simulink model "bf_swarm_generated"  (R2025a)
settings: Solver=ode4  StartTime=0.0  StopTime=60  FixedStep=0.002  RelTol=1e-3
model workspace (MAT data in the model file):
  cfg.N = 3
  cfg.mode = 'paper'
  cfg.T = 60
  cfg.dt = 0.002
  cfg.Ts = 0.01
  cfg.logTs = 0.02
  cfg.visualTs = 0.05
  cfg.visualize = 1
  cfg.pacing = 0
  cfg.receiver = [4; -3; 15]
  cfg.radius = 0.8
  cfg.path.center = [0; 0; 3]
  cfg.path.amplitude = [2.5; 1.5; 0.35]
  cfg.path.period = 40
  cfg.path.ramp = 5
  cfg.path.type = 'figure8'
  cfg.frameSeed = [1; 0; 0]
  cfg.yaw = 0
  cfg.initial.centroidError = [0.15; -0.1; 0.1]
  cfg.initial.formationRotation = [0; 0.209439510239; 0]
  cfg.initial.individualError = 0
  cfg.control.Kp = [2.5; 2.5; 3.5]
  cfg.control.Kd = [2.8; 2.8; 3.2]
  cfg.control.beta = 1.3
  cfg.control.kc = 0.9
  cfg.control.kv = 0.45
  cfg.control.ka = 3.2
  cfg.control.kq = 1
  cfg.control.kPlane = 4
  cfg.control.dPlane = 3
  cfg.control.maxHorizontalAccel = 4
  cfg.control.maxVerticalAccel = 4
  cfg.control.maxTilt = 0.610865238198
  cfg.vehicle.mass = 1
  cfg.vehicle.g = 9.81
  cfg.vehicle.I = [0.015  0  0; 0  0.015  0; 0  0  0.025]
  cfg.vehicle.arm = 0.225
  cfg.vehicle.kT = 1.8e-05
  cfg.vehicle.kQ = 2.7e-07
  cfg.vehicle.motorTau = 0.025
  cfg.vehicle.omegaMax = 620
  cfg.vehicle.drag = [0.12; 0.12; 0.18]
  cfg.vehicle.angularDrag = [0.002; 0.002; 0.003]
  cfg.vehicle.KR = [2.2; 2.2; 1.2]
  cfg.vehicle.Kw = [0.32; 0.32; 0.28]
  cfg.vehicle.bodyRadius = 0.27
  cfg.vehicle.rotorXY = [0.159099025767  -0.159099025767  -0.159099025767  0.159099025767; 0.159099025767  0.159099025767  -0.159099025767  -0.159099025767]
  cfg.vehicle.spin = [1 -1 1 -1]
  cfg.vehicle.B = [1  1  1  1; 0.159099025767  0.159099025767  -0.159099025767  -0.159099025767; -0.159099025767  0.159099025767  0.159099025767  -0.159099025767; 0.015  -0.015  0.015  -0.015]
  cfg.vehicle.Binv = [0.25  1.57134840264  -1.57134840264  16.6666666667; 0.25  1.57134840264  1.57134840264  -16.6666666667; 0.25  -1.57134840264  1.57134840264  16.6666666667; 0.25  -1.57134840264  -1.57134840264  -16.6666666667]
  cfg.vehicle.fMax = 6.9192
  cfg.wind.enabled = 0
  cfg.wind.velocity = [0.8; 0.3; 0]
  cfg.wind.gust = [0.3; 0.2; 0.1]
  cfg.rf.frequency = 138000000
  cfg.rf.c = 299792458
  cfg.rf.powerPerDrone = 0.1
  cfg.rf.noisePower = 1e-13
  cfg.rf.phaseOffsets = [0; 0; 0]
  cfg.rf.enabled = 1
  cfg.rho = [0.8  -0.4  -0.4; 0  0.692820323028  -0.692820323028; 0  0  0]
  cfg.edges = [1  2; 1  3; 2  3]
  cfg.edgeLength = [1.38564064606; 1.38564064606; 1.38564064606]
  cfg.minSeparation = 0.54
  cfg.lambda = 2.17240911594
  cfg.x0 = [0.844904723425  -0.162516209726  -0.232388513699; -0.040298923068  0.542283901867  -0.801984978799; 2.70815410328  3.4602846209  3.13156127581; 0  0  0; 0  0  0; 0  0  0; 1  1  1; 0  0  0; 0  0  0; 0  0  0; 0  0  0; 0  0  0; 0  0  0; 369.120576506  369.120576506  369.120576506; 369.120576506  369.120576506  369.120576506; 369.120576506  369.120576506  369.120576506; 369.120576506  369.120576506  369.120576506]
settings Model: Creator=Pranav R  LastModifiedBy=Pranav R
settings DataIOCC: SaveOutput=off  SignalLogging=off  SaveTime=off

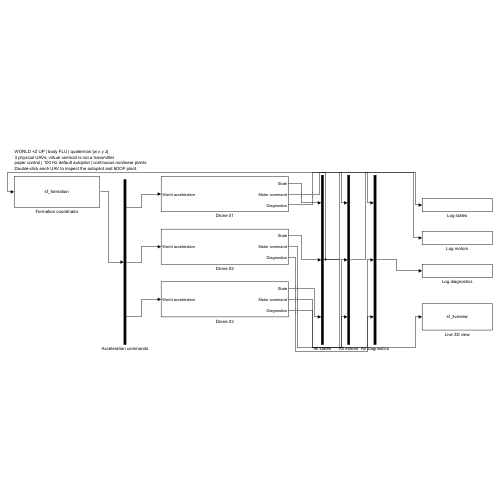
[thumbnail: Simulink's stored preview of the top-level diagram]
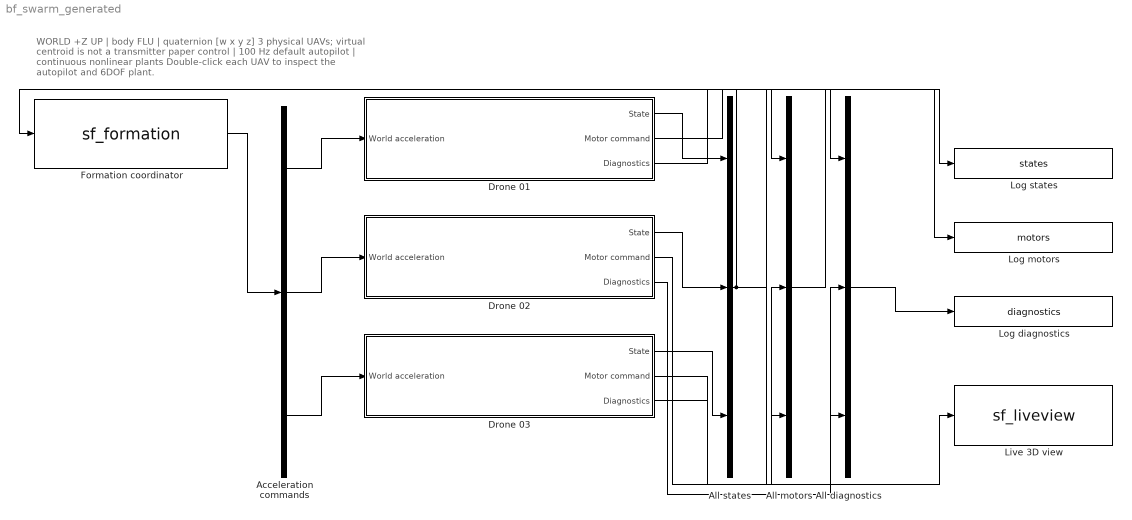
== system bf_swarm_generated ==
  note: WORLD +Z UP | body FLU | quaternion [w x y z]
      | 3 physical UAVs; virtual centroid is not a transmitter
      | paper control | 100 Hz default autopilot | continuous nonlinear plants
      | Double-click each UAV to inspect the autopilot and 6DOF plant.
  Acceleration commands : Demux  Outputs=[3 3 3]
  All diagnostics : Mux  Inputs=3
  All motors : Mux  Inputs=3
  All states : Mux  Inputs=3
  Drone 01 : Subsystem
  Drone 02 : Subsystem
  Drone 03 : Subsystem
  Formation coordinator : M-S-Function  FunctionName=sf_formation  Parameters=cfg
  Live 3D view : M-S-Function  FunctionName=sf_liveview  Parameters=cfg
  Log diagnostics : ToWorkspace  VariableName=diagnostics  SaveFormat=Timeseries  SampleTime=cfg.logTs
  Log motors : ToWorkspace  VariableName=motors  SaveFormat=Timeseries  SampleTime=cfg.logTs
  Log states : ToWorkspace  VariableName=states  SaveFormat=Timeseries  SampleTime=cfg.logTs
  wires:
  Formation coordinator/1 -> Acceleration commands/1
  Acceleration commands/1 -> Drone 01/1(World acceleration)
  Drone 01/1(State) -> All states/1
  Drone 01/2(Motor command) -> All motors/1
  Drone 01/3(Diagnostics) -> All diagnostics/1
  Acceleration commands/2 -> Drone 02/1(World acceleration)
  Drone 02/1(State) -> All states/2
  Drone 02/2(Motor command) -> All motors/2
  Drone 02/3(Diagnostics) -> All diagnostics/2
  Acceleration commands/3 -> Drone 03/1(World acceleration)
  Drone 03/1(State) -> All states/3
  Drone 03/2(Motor command) -> All motors/3
  Drone 03/3(Diagnostics) -> All diagnostics/3
  All states/1 -> Formation coordinator/1, Log states/1, Live 3D view/1
  All motors/1 -> Log motors/1
  All diagnostics/1 -> Log diagnostics/1

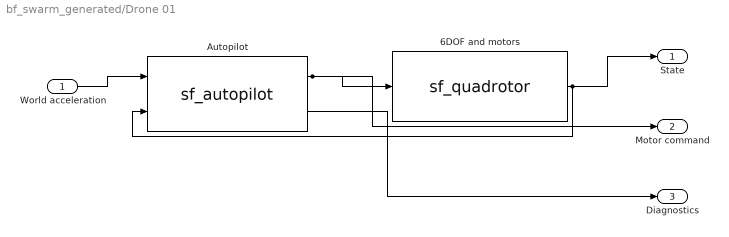
== system bf_swarm_generated/Drone 01 ==
  World acceleration : Inport
  6DOF and motors : M-S-Function  FunctionName=sf_quadrotor  Parameters=cfg,1
  Autopilot : M-S-Function  FunctionName=sf_autopilot  Parameters=cfg
  State : Outport
  Motor command : Outport  Port=2
  Diagnostics : Outport  Port=3
  wires:
  World acceleration/1 -> Autopilot/1
  Autopilot/1 -> 6DOF and motors/1, Motor command/1
  6DOF and motors/1 -> Autopilot/2, State/1
  Autopilot/2 -> Diagnostics/1

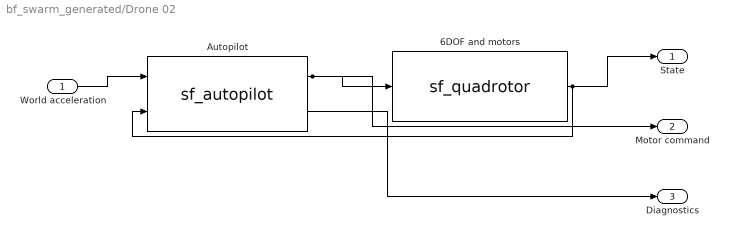
== system bf_swarm_generated/Drone 02 ==
  World acceleration : Inport
  6DOF and motors : M-S-Function  FunctionName=sf_quadrotor  Parameters=cfg,2
  Autopilot : M-S-Function  FunctionName=sf_autopilot  Parameters=cfg
  State : Outport
  Motor command : Outport  Port=2
  Diagnostics : Outport  Port=3
  wires:
  World acceleration/1 -> Autopilot/1
  Autopilot/1 -> 6DOF and motors/1, Motor command/1
  6DOF and motors/1 -> Autopilot/2, State/1
  Autopilot/2 -> Diagnostics/1

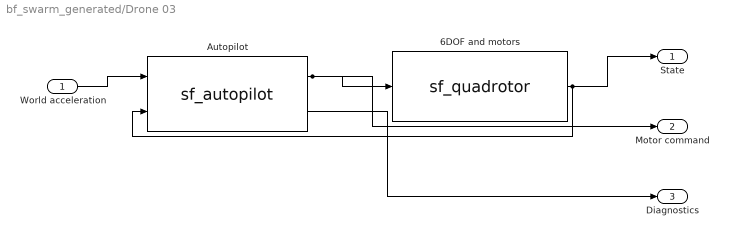
== system bf_swarm_generated/Drone 03 ==
  World acceleration : Inport
  6DOF and motors : M-S-Function  FunctionName=sf_quadrotor  Parameters=cfg,3
  Autopilot : M-S-Function  FunctionName=sf_autopilot  Parameters=cfg
  State : Outport
  Motor command : Outport  Port=2
  Diagnostics : Outport  Port=3
  wires:
  World acceleration/1 -> Autopilot/1
  Autopilot/1 -> 6DOF and motors/1, Motor command/1
  6DOF and motors/1 -> Autopilot/2, State/1
  Autopilot/2 -> Diagnostics/1
